simulink model "es1_sim"  (R2019a)
settings: Solver=VariableStepAuto  StartTime=0.0  StopTime=10.0  RelTol=1e-3
values from neighbouring files (symbols this model uses):
  Cd = c2d(C,Tc,'tustin')    [ES1.m]
  G = tf(num,den)    [ES1.m]
  Tc = 0.001    [ES1.m]
settings Model: Creator=lezione  LastModifiedBy=lezione

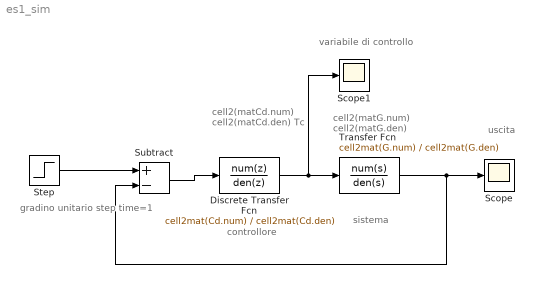
== system es1_sim ==
  note: gradino unitario
      | step time=1
  note: sistema
  note: controllore
  note: variabile di controllo
  note: uscita
  note: cell2(matCd.num)
      | cell2(matCd.den)
      | Tc
  note: cell2(matG.num)
      | cell2(matG.den)
  Discrete Transfer Fcn : DiscreteTransferFcn  Numerator=cell2mat(Cd.num)  Denominator=cell2mat(Cd.den)  SampleTime=Tc
  Scope : Scope
  Scope1 : Scope
  Step : Step  SampleTime=0
  Subtract : Sum  Inputs=+-
  Transfer Fcn : TransferFcn  Numerator=cell2mat(G.num)  Denominator=cell2mat(G.den)
  wires:
  Discrete Transfer Fcn/1 -> Scope1/1, Transfer Fcn/1
  Transfer Fcn/1 -> Subtract/2, Scope/1
  Step/1 -> Subtract/1
  Subtract/1 -> Discrete Transfer Fcn/1
